simulink model "Linearization2"  (R2022a)
settings: Solver=VariableStepAuto  StartTime=0.0  StopTime=10.0  RelTol=1e-3
undefined symbols (not defined in the file): Aactuator, ac, AeroCoeff, ControlAllocation, DUmax, DUmin, EngineTable, F, fcs, ft, g, hground, IC, kg, LandingGear, Light, LPmethod, m, MIL, Mode_deflection_aileron, Mode_deflection_elevator, Mode_deflection_rudder, Mode_deflection_TVC_y, Mode_deflection_TVC_z, N, Ninv_2nozzle, Ninv_no_nozzle, PIController, s, Sensor, slug, state0, sysID_DAQ, sysID_OBES, Umax_2nozzle, Umax_no_nozzle, Umin_2nozzle, Umin_no_nozzle, WMM2020
libraries: aerolibconvert2 x19, slpidlib x6, simulink x6, sharedutil x4, aerolibatmos2 x3, aerolibwind2 x3, aerolibbdyn x3, aerolibgravity2 x2, sharedtransform x1
(part 9 of 9)

== matlab function Linearization2/F-16 Vehicle Systems Model/Vehicle/6DOF (Quaternion)/MATLAB Function ==
  data: dxdt output; xu input; Fxyz input; Mxyz input; AeroFM input; Txyz input; LGxyz input; m input; Ix input; Iy input; Iz input; Ixz input; Heng input; g input
function dxdt = odedot_simulink_TVC_final(xu, Fxyz, Mxyz, AeroFM, Txyz,LGxyz,m,Ix,Iy,Iz,Ixz,Heng,g)
%% Define state 
% 用不到
% npos = xu(1);  %(ft)
% epos = xu(2);  %(ft)
% alt  = xu(3);   %(ft)
%---------------------------Quateration-----------------------
q0 = xu(4);
q1 = xu(5);
q2 = xu(6);
q3 = xu(7);
%--------------------------------------------------
% U = xu(8);%(ft/s)
% V = xu(9);%(ft/s)
% W = xu(10);%(ft/s)

% vt = xu(8);%(ft/s)
% alpha = xu(9);%(rad)****
% beta = xu(10);%(rad)****
P = xu(8);%(rad/s)
Q = xu(9);%(rad/s)
R = xu(10);%(rad/s)

alpha = xu(11);
beta = xu(12);
mu = xu(13);
vt = xu(14);
chi = xu(15);
gamma = xu(16);

%-------------------------control----------------------
% 推力
Tx   = Txyz(1);
Ty   = Txyz(2);
Tz   = Txyz(3);
% Mx_T = xu(20);
% My_T = xu(21);
% Mz_T = xu(22);

% 用不到
% T = xu(23);%(lbs)
% el = xu(24);%(deg)
% ail = xu(25);%(deg)
% rud = xu(26);%(deg)
% delta_z = xu(27);%(deg)
% delta_y = xu(28);%(deg)

%% ISP
% qbar = xu(29);
%% Aerodynamic coefficient
% CXT = xu(30);
% CYT = xu(31);
% CZT = xu(32);
% CLT = xu(33);
% CMT = xu(34);
% CNT = xu(35);

% lef = xu(36);%(deg)



%% Dimension Convert
% r2d = 180/pi;    %rad to deg
% d2r = pi/180;    %deg to rad
% m2f = 3.2808399; %meter to ft. Same as m/s to ft/s
% f2m = 0.3048;    %ft to meter. Same as ft/s to m/s
%
% theta = asin((2*q0*q2)-(2*q3*q1));%rad
% psi = atan((2*(q0*q3+q1*q2))/(q0^2+q1^2-q2^2-q3^2));%rad
% phi = atan((2*(q0*q1+q2*q3))/(q0^2-q1^2-q2^2+q3^2));%rad

%% Aircraft parameters
% g = 32.17;       %gravity, ft/s^2
% m  = 636.94;     %mass, slugs
% B  = 30.0;       %span, ft
% S = 300.0;       %planform area, ft^2
% cbar = 11.32;    %mean aero chord, ft
% x_cg_ref = 0.35;     %reference center of gravity as a fraction of cbar
% x_cg = 0.30;      %center of gravity as a fraction of cbar.
% Heng = 0.0;      %turbine momentum along roll axis.

% Ix = 9496.0;     %slug-ft^2
% Iy = 55814.0;    %slug-ft^2
% Iz = 63100.0;    %slug-ft^2
% Ixz = 982.0;     %slug-ft^2
%-------------------------Abbreviation----------------------
sa = sin(alpha);  %sin(alpha)
ca = cos(alpha);  %cos(alpha)
sb = sin(beta);  %sin(beta)
cb = cos(beta);  %cos(beta)
tb = tan(beta);  %tan(beta)
% st = sin(theta);  %cos(beta)
% ct = cos(theta);
% tt = tan(theta);
% sphi = sin(phi);
% cphi = cos(phi);
% spsi = sin(psi);
% cpsi = cos(psi);

% %% Calculate Aerdynamic Coefficients
% % [alpha,beta,ele,ail,rud,lef,tot_V,p,q,r]
% Aero_coe = [alpha*r2d,beta*r2d,el,ail,rud,lef,vt,P,Q,R];       %Simulink type
% [Aerodynamic_coe] = Aerodynamic_coefficient(Aero_coe);   %[Cx_tot Cy_tot Cz_tot Cl_tot Cm_tot Cn_tot];
% %% Calculate ISP
% h = alt*f2m;   %ISP code h is meter! Must changed(alt:feet)
% ISP_output = Standard_Atmosphere1(h); %[T(k),a(m/s),P(Pa),rho(kg/m^3),g(m/s^2),mu]
% % Mach = vt/(ISP_output(2)*m2f);
% qbar = 0.5*( 0.00194032033*ISP_output(4) )*(vt^2);
% % g = ISP_output(5)*m2f
%% Lift Drag Side force
% X = qbar*S*CXT;
% Y = qbar*S*CYT;
% Z = qbar*S*CZT;
X = AeroFM(1);
Y = AeroFM(2);
Z = AeroFM(3);

D = -X*ca*cb - Y*sb - Z*sa*cb;
Y_bar = -X*ca*sb + Y*cb - Z*sa*sb;
L = X*sa - Z*ca;
%% qnorm
QQ = q0^2+q1^2+q2^2+q3^2;
q0 = q0/sqrt(QQ);
q1 = q1/sqrt(QQ);
q2 = q2/sqrt(QQ);
q3 = q3/sqrt(QQ);
%% Equations
U = vt*ca*cb;  % directional velocities.
V = vt*sb;
W = vt*sa*cb;
%% LandingGear force
f = LGxyz(1); % Friction force
N = LGxyz(3); % Normal force
%-------------------------Navigation Equations----------------------
% xdot1 = U*(ct*cpsi) + V*(sphi*cpsi*st - cphi*spsi) +  W*(cphi*st*cpsi + sphi*spsi);%nposdot
% xdot2 = U*(ct*spsi) +  V*(sphi*spsi*st + cphi*cpsi) +  W*(cphi*st*spsi - sphi*cpsi);%eposdot
% xdot3 = -U*st + V*(sphi*ct) + W*(cphi*ct);%altdot
xdot1 = U*(q0*q0+q1*q1-q2*q2-q3*q3) + 2*V*(q1*q2-q0*q3) +  2*W*(q1*q3+q0*q2);%nposdot
xdot2 = 2*U*(q1*q2+q0*q3) +  V*(q0*q0-q1*q1+q2*q2-q3*q3) +  2*W*(q2*q3-q0*q1);%eposdot
xdot3 = 2*U*(q1*q3-q0*q2) + 2*V*(q2*q3+q0*q1) + W*(q0*q0-q1*q1-q2*q2+q3*q3);%altdot
%------------------------- Kinematic Equations----------------------
% xdot4 = P + tt*(Q*sphi + R*cphi);%phidot
% xdot5 = Q*cphi - R*sphi;%theta dot
% xdot6 = (Q*sphi + R*cphi)/ct;%psidot
xdot4 = -0.5*(P*q1+Q*q2+R*q3);
xdot5 = -0.5*(-P*q0-R*q2+Q*q3);
xdot6 = -0.5*(-Q*q0+R*q1-P*q3);
xdot7 = -0.5*(-R*q0-Q*q1+P*q2);
%-------------------------Compute Udot,Vdot, Wdot----------------------
% Udot = R*V - Q*W - g*st + qbar*S*CXT/m + T/m;
% Vdot = P*W - R*U + g*ct*sphi + qbar*S*CYT/m;
% Wdot = Q*U - P*V + g*ct*cphi + qbar*S*CZT/m;

% Udot = R*V - Q*W + 2*g*(q1*q3)-2*g*(q0*q2) + qbar*S*CXT/m + T/m;
% Vdot = P*W - R*U + 2*g*(q2*q3)+2*g*(q0*q1) + qbar*S*CYT/m;
% Wdot = Q*U - P*V + (q0*q0-q1*q1-q2*q2+q3*q3)*g + qbar*S*CZT/m;

% xdot8 = (U*Udot + V*Vdot + W*Wdot)/vt;%vt_dot
% 
% xdot9 = (U*Wdot - W*Udot)/(U*U + W*W);%alpha_dot
% xdot10 = (Vdot*vt - V*xdot8)/(vt*vt*cb);%beta_dot
%-------------------------Compute Pdot, Qdot, and Rdot----------------------
% L_tot = CLT*qbar*S*B;    %get moments from coefficients */
% M_tot = CMT*qbar*S*cbar;
% N_tot = CNT*qbar*S*B;
% L_tot = AeroFM(4);
% M_tot = AeroFM(5);
% N_tot = AeroFM(6);
% 
% Mx = L_tot+Mx_T;
% My = M_tot+My_T;
% Mz = N_tot+Mz_T;

Mx = Mxyz(1);
My = Mxyz(2);
Mz = Mxyz(3);

denom = Ix*Iz - Ixz*Ixz;


xdot8 =  (Iz*Mx + Ixz*Mz - (Iz*(Iz-Iy)+Ixz*Ixz)*Q*R + Ixz*(Ix-Iy+Iz)*P*Q + Ixz*Q*Heng)/denom;     % Pdot
xdot9 = (My + (Iz-Ix)*P*R - Ixz*(P*P-R*R) - R*Heng)/Iy;                                           % Qdot
xdot10 = (Ix*Mz + Ixz*Mx + (Ix*(Ix-Iy)+Ixz*Ixz)*P*Q - Ixz*(Ix-Iy+Iz)*Q*R +  Ix*Q*Heng)/denom;     % Rdot
%% alpha beta mu vt chi gamma

xdot11 = Q-tb*(P*ca+R*sa)+ ( ( -L+m*g*cos(gamma)*cos(mu) )+ ( -Tx*sa+Tz*ca ) + ( N*cos(gamma)*cos(mu) ) + ( f*(sin(chi)*sin(mu)+cos(chi)*cos(mu)*sin(gamma)) )) /(m*vt*cb);
% xdot14 = -sa/(vt*cb)*Udot + ca/(vt*cb)*Wdot;

xdot12 = -R*ca + P*sa + ( Y_bar*cb+m*g*cos(gamma)*sin(mu) -Tx*sb*ca + Ty*cb - Tz*sb*sa + N*cos(gamma)*sin(mu) - f*(cos(mu)*sin(chi)-cos(chi)*sin(gamma)*sin(mu)) ) / (m*vt);
% xdot15 = (-sb*ca/vt)*Udot + (cb/vt)*Vdot + (-sb*sa/vt)*Wdot;

xdot13 = ( P*ca+R*sa ) / cb + ( L / ( m*vt ) )*( tan(gamma)*sin(mu)+tb ) + ( (Y_bar + Ty) / (m*vt) )*tan(gamma)*cos(mu)*cb+...
    + (-g/vt)*cos(gamma)*cos(mu)*tb + (Tx*sa - Tz*ca)*( tan(gamma)*sin(mu)+tb ) / (m*vt) - (Tx*ca + Tz*sa)*( tan(gamma)*cos(mu)*sb ) / (m*vt)+...
    - N*tb*cos(gamma)*cos(mu) / (m*vt) - f*( cos(mu)*cos(chi)*sin(gamma)*tb + sin(chi)*tan(gamma) + sin(chi)*tb*sin(mu) ) / (m*vt);

% vt_dot
xdot14 = (-D + Y_bar*sb -m*g*sin(gamma) + Tx*cb*ca + Ty*sb + Tz*cb*sa - N*sin(gamma) + f*cos(chi)*cos(gamma) ) / (m);
% xdot17 = cb*ca*Udot + sb*Vdot + cb*sa*Wdot;

% chi_dot
xdot15 = ( L*sin(mu) + Y_bar*cos(mu)*cb + Tx*( sin(mu)*sa - cos(mu)*sb*ca) + Ty*(cos(mu)*cb) -Tz*( cos(mu)*sb*sa+sin(mu)*ca ) - f*sin(chi) ) / ( m*vt*cos(gamma) );

% gamma_dot
xdot16 = ( L*cos(mu) - Y_bar*sin(mu)*cb - m*g*cos(gamma) + Tx* ( sin(mu)*sb*ca + cos(mu)*sa ) -Ty*(sin(mu)*cb) + Tz*( sin(mu)*sb*sa-cos(mu)*ca ) - N*cos(gamma) - f*cos(chi)*sin(gamma) ) / (m*vt);


%%
dxdt = zeros(16,1);  % 定義局部變數。 The first assignment to a local variable determines its class.
dxdt(1) = xdot1;
dxdt(2) = xdot2;
dxdt(3) = xdot3;
dxdt(4) = xdot4;
dxdt(5) = xdot5;
dxdt(6) = xdot6;
dxdt(7) = xdot7;
dxdt(8) = xdot8;
dxdt(9) = xdot9;
dxdt(10) = xdot10;

dxdt(11) = xdot11;
dxdt(12) = xdot12;
dxdt(13) = xdot13;
dxdt(14) = xdot14;
dxdt(15) = xdot15;
dxdt(16) = xdot16;

end

== matlab function Linearization2/F-16 Vehicle Systems Model/Vehicle/6DOF (Quaternion)/MATLAB Function2 ==
  data: p input; q input; r input; alpha input; beta input; mu input; vt input; gamma input; an output; ay output; alpha_dot input; beta_dot input; Vt_dot input; g input
function [an,ay] = load_factor(p,q,r,alpha,beta, mu,vt,gamma, alpha_dot, beta_dot, Vt_dot, g)
% p =xu(1);
% q = xu(2);
% r = xu(3);
% alpha =xu(4);
% beta = xu(5);
% mu = xu(6);
% vt = xu(7);
% % chi = xu(8);
% gamma = xu(9);
% g = 32.17;

cb = cos(beta);
ca = cos(alpha);
sb = sin(beta);
sa = sin(alpha);
the = alpha + gamma;
phi = mu;


u = vt*cb*ca;
v = vt*sb;
w = v*cb*sa;

wdot = Vt_dot*cb*ca - alpha_dot*vt*cb*ca + beta_dot*vt*sb*sa;
Vt_dot_s = Vt_dot*sb + beta_dot*vt*cb; 


an = (q*u - p*v + g*cos(the)*cos(phi)-wdot)/g;
ay = (-p*w + r*u - g*cos(the)*sin(phi) + Vt_dot_s)/g;


% anz = an;
% anz = [an ay];
end

== matlab function Linearization2/F-16 Vehicle Systems Model/pqr NDI Controller/ f1 ==
  data: f1 output size=3; moments input; pqr input; Ix input; Iy input; Iz input; Ixz input
function f1 = NDI_f_fast(moments, pqr,Ix,Iy,Iz,Ixz)
p = pqr(1);
q = pqr(2);
r = pqr(3);
L_hat = moments(1);
M_hat = moments(2);
N_hat = moments(3);

f1 = zeros(3,1);
f1(1) = (Iz*L_hat + Ixz*N_hat) / (Ix*Iz - Ixz^2) + ( Ixz*(Ix - Iy + Iz)*p*q + (Iz*(Iy - Iz) - Ixz^2)*q*r ) / (Ix*Iz - Ixz^2);
f1(2) = M_hat / Iy + ((Iz - Ix)*p*r + Ixz*(r^2-p^2)) / Iy;
f1(3) = (Ixz*L_hat + Ix*N_hat) / (Ix*Iz - Ixz^2) + ( (Ix*(Ix - Iy) + Ixz^2)*p*q - Ixz*(Ix - Iy + Iz)*q*r ) / (Ix*Iz - Ixz^2);
end

== stateflow chart Linearization2/F-16 Vehicle Systems Model/pqr NDI Controller/Control Allocation/Chart ==
  state DA
  state TakeOff_Landing
  state HighManeuverability
  state Cruise
  state Penetration
  note: 需有一個訊號[被雷達鎖定、飛彈來襲]，
      | 解除突防，跳入直接幾何法(接戰模式)
  (default) -> DA : {CA=4;}
  DA -> (junction 92)
  (junction 110) -> DA
  (junction 92) -> DA [order 3] : [switchhh==0]{CA=4;}
  (junction 92) -> Penetration [order 2] : [switchhh==1]{CA=8;}
  (junction 92) -> (junction 98) [order 1] : [switchhh==0]
  TakeOff_Landing -> (junction 110)
  HighManeuverability -> (junction 110)
  Cruise -> (junction 110)
  Penetration -> (junction 110) : [switchhh==0]
  (junction 98) -> TakeOff_Landing [order 1] : [Vt<300&&altitude<1000]{CA=7;}
  (junction 98) -> (junction 102) [order 2]
  (junction 102) -> HighManeuverability [order 1] : [alpha>35]{CA=9;}
  (junction 102) -> (junction 106) [order 2]
  (junction 106) -> Cruise : [Vt_dot<5&&altitude_dot<5]{CA=6;}
  data: CA output; alpha input; Vt input; altitude input; Vt_dot input; altitude_dot input; switchhh input

== matlab function Linearization2/F-16 Vehicle Systems Model/pqr NDI Controller/Control Allocation/Pseudo_inverses_ShunYuanChang2019/Control Allocation ==
  data: u_bar output; y_bar input; g1 input; N input
function u_bar = NDI(y_bar, g1, N)
% 聯動式(控制配置)

% 提醒：MATLAB Function模塊的 *.m檔裡面，不能使用disp( ) 打印輸出中文字，不然會回報莫名其妙的錯誤 (port widths or dimensions 錯誤 )
% disp('run Pseudo_inverses_ShunYuanChang2019')

% 權重矩陣N 改由 PreLoadFcn.m 做設定和載入

pseudo_inv_gt_f = pinv(g1*N);
u_bar = N*pseudo_inv_gt_f*y_bar;

% right_aileron  = u_bar(1);
% left_aileron   = u_bar(2)
% right_elevator = u_bar(3);
% left_elevator  = u_bar(4);
% rudder         = u_bar(5);  
% TVC_ry         = u_bar(6);  勁豪跟舜淵的 TVC_Y TVC_Z 定義相反
% TVC_rz         = u_bar(7);
% TVC_ly         = u_bar(6);
% TVC_lz         = u_bar(7);

end
